simulink model "furuta_pendulum_d"  (R2016a)
settings: Solver=VariableStepAuto  StartTime=0.0  StopTime=10.0  RelTol=1e-3
undefined symbols (not defined in the file): alpha, beta, delta, dq0, gamma, h, la, lp, q0
settings Model: Creator=mgreiff  LastModifiedBy=mgreiff
settings DataIOCC: LimitDataPoints=on
settings DebuggingCC: AllowSymbolicDim=off
settings ModelReferenceCC: PropagateSignalLabelsOutOfModel=off
settings GRTTargetCC: GeneratePreprocessorConditionals=Use local settings

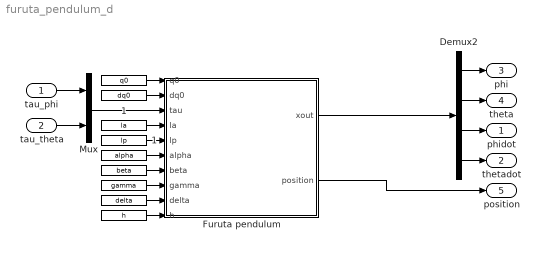
== system furuta_pendulum_d ==
  tau_phi : Inport  PortDimensions=1
  tau_theta : Inport  Port=2  PortDimensions=1
  " " : Constant  Value=alpha
  "  " : Constant  Value=beta
  "   " : Constant  Value=gamma
  "    " : Constant  Value=delta
  "     " : Constant  Value=h
  "      " : Constant  Value=q0
  "        " : Constant  Value=dq0
  "  1" : Constant  Value=lp
  " 1" : Constant  Value=la
  Demux2 : Demux
  Furuta pendulum : MATLAB Function  TreatAsAtomicUnit=on  SystemSampleTime=h
  Mux : Mux  Inputs=2
  "phidot " : Outport  PortDimensions=1
  thetadot : Outport  Port=2  PortDimensions=1
  phi : Outport  Port=3  PortDimensions=1
  theta : Outport  Port=4  PortDimensions=1
  "position " : Outport  Port=5  PortDimensions=3
  wires:
  tau_phi/1 -> Mux/1
  tau_theta/1 -> Mux/2
  Mux/1 -> Furuta pendulum/3(tau)
  " "/1 -> Furuta pendulum/6(alpha)
  "  "/1 -> Furuta pendulum/7(beta)
  "   "/1 -> Furuta pendulum/8(gamma)
  "    "/1 -> Furuta pendulum/9(delta)
  Demux2/4 -> thetadot/1
  Demux2/3 -> "phidot "/1
  Demux2/2 -> theta/1
  Demux2/1 -> phi/1
  " 1"/1 -> Furuta pendulum/4(la)
  "  1"/1 -> Furuta pendulum/5(lp)
  Furuta pendulum/2(position) -> "position "/1
  "     "/1 -> Furuta pendulum/10(h)
  "      "/1 -> Furuta pendulum/1(q0)
  "        "/1 -> Furuta pendulum/2(dq0)
  Furuta pendulum/1(xout) -> Demux2/1

== matlab function furuta_pendulum_d/Furuta pendulum ==
  data: q0 input; dq0 input; tau input; la input; lp input; xout output; alpha input; beta input; gamma input; delta input; position output; h input
function [xout, position]= fcn(q0, dq0, tau, la, lp, alpha, beta, gamma, delta, h)
%#codegen
persistent x;
if isempty(x)
    x = [q0; dq0];
end

% State and control signal extraction
phi    = x(1);
theta  = x(2);
dphi   = x(3);
dtheta = x(4);
u = tau;

% Precomputation
cp = cos(phi);
sp = sin(phi);
ct = cos(theta);
st = sin(theta);

% Form conttinuous time system
M = [alpha + beta*(st.^2), gamma * ct;
     gamma * ct          , beta     ];
C = [ beta * ct * st * dtheta, beta * ct * st * dphi - gamma * st * dtheta;
     -beta * ct * st * dphi  , 0                                         ];
G = [0; -delta * st];

Z2 = zeros(2);
I2 = eye(2);
Ac = [Z2,   I2;
      Z2, -M\C];
Bc = [Z2;
      M\I2];
Gc = [0;0;-M\G];

% Discretize system
expMat = expm(h*[Ac, Bc, Gc; zeros(3,7)]);
Ad = expMat(1:4,1:4);
Bd = expMat(1:4,5:6); 
Gd = expMat(1:4,7);

% Predict forward
x = Ad*x + Bd*u + Gd;
xout = x;

% Compute position in global coordinates for debugging
px = la * cp - lp * sp * st;
py = la * sp + lp * cp * st;
pz = lp * ct;
position = [px;py;pz];
end
